simulink library "WECSim_Lib_Controllers"  (R2021b)
settings: Solver=ode45  StartTime=0.0  StopTime=10.0  RelTol=1e-3  EnableMultiTasking=on
undefined symbols (not defined in the file or in its folder): controller, controlSim, simu
settings Model: RequirementInfo="{}  %GIDa_42666abb_d6d9_408c_ae24_f6520282b61c"  Creator=sor  LastModifiedBy=jtgrasb
settings SolverCC: AlgebraicLoopSolver=TrustRegion
settings DataIOCC: LimitDataPoints=on  SaveFormat=Array  ReturnWorkspaceOutputs=off
settings OptimizationCC: LifeSpan=inf
settings DebuggingCC: SolverPrmCheckMsg=warning  AllowSymbolicDim=off  SFUnexpectedBacktrackingDiag=warning  SFNoUnconditionalDefaultTransitionDiag=warning  SFExecutionAtInitializationDiag=none  SFMachineParentedDataDiag=warning  ArithmeticOperatorsInVariantConditions=warning
settings HardwareCC: ProdBitPerPointer=32  ProdBitPerSizeT=32  ProdBitPerPtrDiffT=32  ProdLargestAtomicFloat=None  ProdIntDivRoundTo=Undefined  ProdEndianess=Unspecified  ProdWordSize=32  ProdHWDeviceType=32-bit Generic
settings ModelReferenceCC: PropagateSignalLabelsOutOfModel=off
settings SFSimCC: SimUseLocalCustomCode=off  CustomCodeUndefinedFunction=UseInterfaceOnly
settings RTWCC: RTWUseLocalCustomCode=off
settings CodeAppCC: StateflowObjectComments=on
settings GRTTargetCC: TargetLangStandard=C89/C90 (ANSI)
settings ConfigComp: CovMetricSettings=dw  CovSaveCumulativeToWorkspaceVar=on  CovSaveSingleToWorkspaceVar=on  CovExternalEMLEnable=off  CovSFcnEnable=off

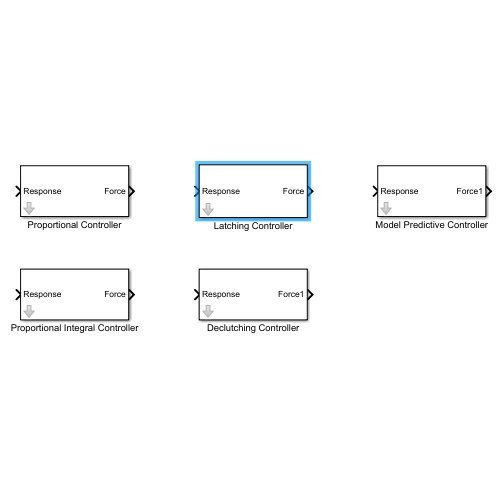
[thumbnail: Simulink's stored preview of the top-level diagram]
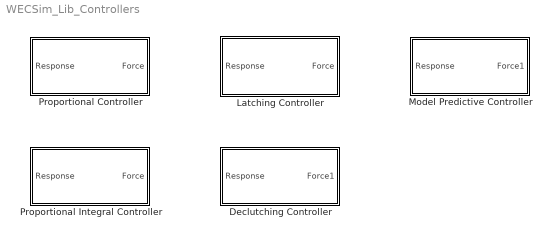
== system WECSim_Lib_Controllers ==
  Declutching Controller : Subsystem  mask{controller=controller(1), InputFiletext=Use WEC-Sim input file to define Latching Controller parameters, Kp=0, Ki=0, declutchTime=0}
      mask prompts: controller "Controller Name:"; Kp "Proportional gain (damping) [Ns/m]"; Ki "Integral gain (stiffness) [N/m]"; declutchTime "Declutching Time [s]"
      mask init:
      | if exist('controller','var')
      |     h=[gcb '/To Workspace'];
      |     responseName=['controller' num2str(controller.number) '_out'];
      |     set_param(h,'VariableName',responseName);
      | end
      | clear h responseName
      mask DialogControl InputFileGroup Prompt: Input File
      mask DialogControl CustomParameterGroup Prompt: Custom Parameters
      mask DialogControl DCParameters Prompt: Declutching Controller Parameters
  Latching Controller : Subsystem  mask{controller=controller(1), InputFiletext=Use WEC-Sim input file to define Latching Controller parameters, Kp=0, Ki=0, latchTime=0}
      mask prompts: controller "Controller Name"; Kp "Proportional gain (damping) [Ns/m]"; Ki "Integral gain (stiffness) [N/m]"; latchTime "Latching Time [s]"
      mask init:
      | if exist('controller','var')
      |     h=[gcb '/To Workspace'];
      |     responseName=['controller' num2str(controller.number) '_out'];
      |     set_param(h,'VariableName',responseName);
      | end
      | clear h responseName
      mask DialogControl InputFileGroup Prompt: Input File
      mask DialogControl CustomParameterGroup Prompt: Custom Parameters
      mask DialogControl LCParameters Prompt: Latching Controller Parameters
  Model Predictive Controller : Subsystem  mask{controller=controller(1), InputFiletext=Use WEC-Sim input file to define Latching Controller parameters, Kp=0, Ki=0, declutchTime=0}
      mask prompts: controller "Controller Name:"; Kp "Proportional gain (damping) [Ns/m]"; Ki "Integral gain (stiffness) [N/m]"; declutchTime "Declutching Time [s]"
      mask init:
      | if exist('controller','var')
      |     h=[gcb '/To Workspace'];
      |     responseName=['controller' num2str(controller.number) '_out'];
      |     set_param(h,'VariableName',responseName);
      | end
      | clear h responseName
      mask DialogControl InputFileGroup Prompt: Input File
      mask DialogControl CustomParameterGroup Prompt: Custom Parameters
      mask DialogControl DCParameters Prompt: Declutching Controller Parameters
  Proportional Controller : Subsystem  mask{controller=controller(1), InputFiletext=Use WEC-Sim input file to define Latching Controller parameters, Kp=0}
      mask prompts: controller "Controller Name:"; Kp "Proportional gain (damping) [Ns/m]"
      mask init:
      | if exist('controller','var')
      |     h=[gcb '/To Workspace'];
      |     responseName=['controller' num2str(controller.number) '_out'];
      |     set_param(h,'VariableName',responseName);
      | end
      | clear h responseName
      mask DialogControl InputFileGroup Prompt: Input File
      mask DialogControl CustomParameterGroup Prompt: Custom Parameters
      mask DialogControl PCParameters Prompt: Proportional Controller Parameters
  Proportional Integral Controller : Subsystem  mask{controller=controller(1), InputFiletext=Use WEC-Sim input file to define Latching Controller parameters, Kp=0, Ki=0}
      mask prompts: controller "Controller Name:"; Kp "Proportional gain (damping) [Ns/m]"; Ki "Integral gain (stiffness) [N/m]"
      mask init:
      | if exist('controller','var')
      |     h=[gcb '/To Workspace'];
      |     responseName=['controller' num2str(controller.number) '_out'];
      |     set_param(h,'VariableName',responseName);
      | end
      | clear h responseName
      mask DialogControl InputFileGroup Prompt: Input File
      mask DialogControl CustomParameterGroup Prompt: Custom Parameters
      mask DialogControl PICParameters Prompt: Proportional Integral Controller Parameters

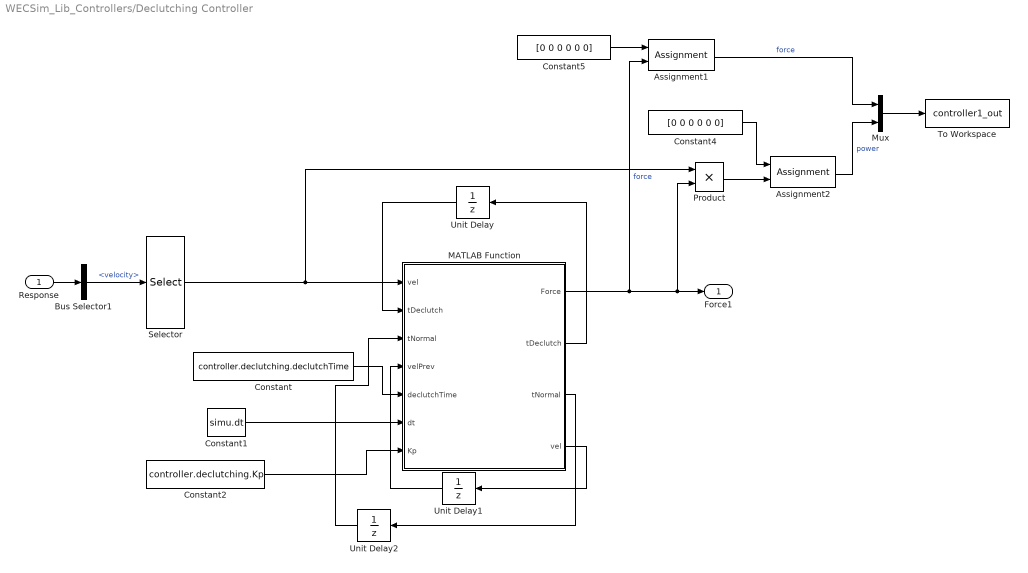
== system WECSim_Lib_Controllers/Declutching Controller ==
  Response : Inport
  Assignment1 : Assignment  IndexOptions=Index vector (dialog)  Indices=3  OutputSizes=1
  Assignment2 : Assignment  IndexOptions=Index vector (dialog)  Indices=3  OutputSizes=1
  Bus Selector1 : BusSelector  OutputSignals=velocity
  Constant : Constant  Value=controller.declutching.declutchTime
  Constant1 : Constant  Value=simu.dt
  Constant2 : Constant  Value=controller.declutching.Kp
  Constant4 : Constant  Value=[0 0 0 0 0 0]
  Constant5 : Constant  Value=[0 0 0 0 0 0]
  MATLAB Function : MATLAB Function  TreatAsAtomicUnit=on
  Mux : Mux  Inputs=2
  Product : Product
  Selector : Selector  InputPortWidth=6  IndexOptions=Index vector (dialog)  Indices=3  OutputSizes=1
  To Workspace : ToWorkspace  VariableName=controller1_out  SaveFormat=Structure With Time  SampleTime=simu.dtOut
  Unit Delay : UnitDelay  SampleTime=-1  HasFrameUpgradeWarning=on
  Unit Delay1 : UnitDelay  SampleTime=-1  HasFrameUpgradeWarning=on
  Unit Delay2 : UnitDelay  SampleTime=-1  HasFrameUpgradeWarning=on
  Force1 : Outport
  wires:
  Bus Selector1/1 -> Selector/1  "<velocity>"
  MATLAB Function/4(vel) -> Unit Delay1/1
  Unit Delay2/1 -> MATLAB Function/3("tNormal ")
  Constant2/1 -> MATLAB Function/7(Kp)
  Unit Delay1/1 -> MATLAB Function/4(velPrev)
  MATLAB Function/3(tNormal) -> Unit Delay2/1
  Constant/1 -> MATLAB Function/5(declutchTime)
  Unit Delay/1 -> MATLAB Function/2("tDeclutch ")
  Constant1/1 -> MATLAB Function/6(dt)
  MATLAB Function/2(tDeclutch) -> Unit Delay/1
  Response/1 -> Bus Selector1/1
  Constant4/1 -> Assignment2/1
  Assignment2/1 -> Mux/2  "power"
  Product/1 -> Assignment2/2
  MATLAB Function/1(Force) -> Force1/1, Product/2, Assignment1/2  "force"
  Assignment1/1 -> Mux/1  "force"
  Mux/1 -> To Workspace/1
  Selector/1 -> Product/1, MATLAB Function/1("vel ")
  Constant5/1 -> Assignment1/1

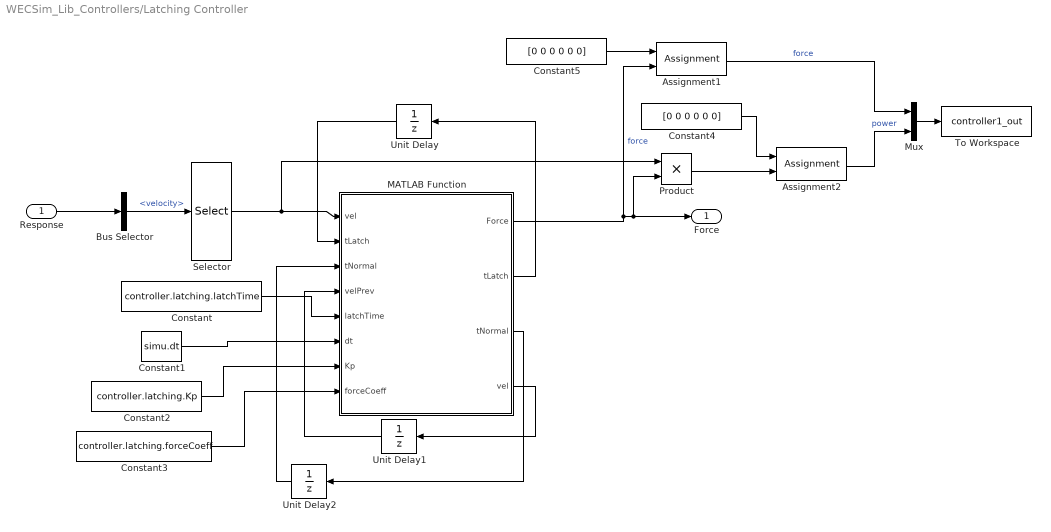
== system WECSim_Lib_Controllers/Latching Controller ==
  Response : Inport
  Assignment1 : Assignment  IndexOptions=Index vector (dialog)  Indices=3  OutputSizes=1
  Assignment2 : Assignment  IndexOptions=Index vector (dialog)  Indices=3  OutputSizes=1
  Bus Selector : BusSelector  OutputSignals=velocity
  Constant : Constant  Value=controller.latching.latchTime
  Constant1 : Constant  Value=simu.dt
  Constant2 : Constant  Value=controller.latching.Kp
  Constant3 : Constant  Value=controller.latching.forceCoeff
  Constant4 : Constant  Value=[0 0 0 0 0 0]
  Constant5 : Constant  Value=[0 0 0 0 0 0]
  MATLAB Function : MATLAB Function  TreatAsAtomicUnit=on
  Mux : Mux  Inputs=2
  Product : Product
  Selector : Selector  InputPortWidth=6  IndexOptions=Index vector (dialog)  Indices=3  OutputSizes=1
  To Workspace : ToWorkspace  VariableName=controller1_out  SaveFormat=Structure With Time  SampleTime=simu.dtOut
  Unit Delay : UnitDelay  SampleTime=-1  HasFrameUpgradeWarning=on
  Unit Delay1 : UnitDelay  SampleTime=-1  HasFrameUpgradeWarning=on
  Unit Delay2 : UnitDelay  SampleTime=-1  HasFrameUpgradeWarning=on
  Force : Outport
  wires:
  Constant1/1 -> MATLAB Function/6(dt)
  Response/1 -> Bus Selector/1
  MATLAB Function/3(tNormal) -> Unit Delay2/1
  MATLAB Function/2(tLatch) -> Unit Delay/1
  Unit Delay2/1 -> MATLAB Function/3("tNormal ")
  Unit Delay1/1 -> MATLAB Function/4(velPrev)
  Unit Delay/1 -> MATLAB Function/2("tLatch ")
  Bus Selector/1 -> Selector/1  "<velocity>"
  Constant/1 -> MATLAB Function/5(latchTime)
  Selector/1 -> Product/1, MATLAB Function/1("vel ")
  MATLAB Function/4(vel) -> Unit Delay1/1
  Constant2/1 -> MATLAB Function/7(Kp)
  Constant5/1 -> Assignment1/1
  Mux/1 -> To Workspace/1
  MATLAB Function/1(Force) -> Product/2, Force/1, Assignment1/2  "force"
  Assignment1/1 -> Mux/1  "force"
  Assignment2/1 -> Mux/2  "power"
  Product/1 -> Assignment2/2
  Constant4/1 -> Assignment2/1
  Constant3/1 -> MATLAB Function/8(forceCoeff)

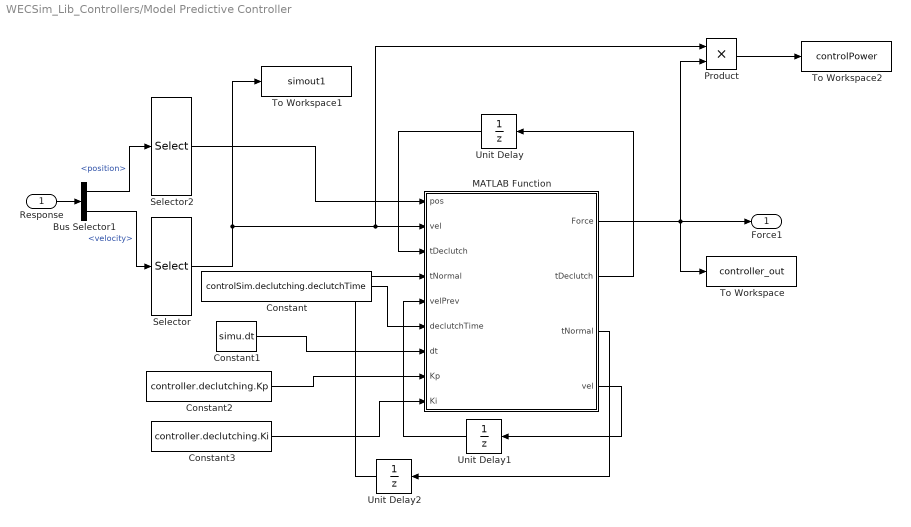
== system WECSim_Lib_Controllers/Model Predictive Controller ==
  Response : Inport
  Bus Selector1 : BusSelector  OutputSignals=position,velocity
  Constant : Constant  Value=controlSim.declutching.declutchTime
  Constant1 : Constant  Value=simu.dt
  Constant2 : Constant  Value=controller.declutching.Kp
  Constant3 : Constant  Value=controller.declutching.Ki
  MATLAB Function : MATLAB Function  TreatAsAtomicUnit=on
  Product : Product
  Selector : Selector  InputPortWidth=6  IndexOptions=Index vector (dialog)  Indices=3  OutputSizes=1
  Selector2 : Selector  InputPortWidth=6  IndexOptions=Index vector (dialog)  Indices=3  OutputSizes=1
  To Workspace : ToWorkspace  VariableName=controller_out  SaveFormat=Timeseries  SampleTime=-1
  To Workspace1 : ToWorkspace  VariableName=simout1  SaveFormat=Timeseries  SampleTime=-1
  To Workspace2 : ToWorkspace  VariableName=controlPower  SaveFormat=Timeseries  SampleTime=-1
  Unit Delay : UnitDelay  SampleTime=-1  HasFrameUpgradeWarning=on
  Unit Delay1 : UnitDelay  SampleTime=-1  HasFrameUpgradeWarning=on
  Unit Delay2 : UnitDelay  SampleTime=-1  HasFrameUpgradeWarning=on
  Force1 : Outport
  wires:
  Response/1 -> Bus Selector1/1
  MATLAB Function/2(tDeclutch) -> Unit Delay/1
  Constant1/1 -> MATLAB Function/7(dt)
  Unit Delay/1 -> MATLAB Function/3("tDeclutch ")
  Constant/1 -> MATLAB Function/6(declutchTime)
  MATLAB Function/3(tNormal) -> Unit Delay2/1
  Constant3/1 -> MATLAB Function/9(Ki)
  Unit Delay1/1 -> MATLAB Function/5(velPrev)
  Constant2/1 -> MATLAB Function/8(Kp)
  MATLAB Function/1(Force) -> To Workspace/1, Force1/1, Product/2
  Unit Delay2/1 -> MATLAB Function/4("tNormal ")
  MATLAB Function/4(vel) -> Unit Delay1/1
  Bus Selector1/2 -> Selector/1  "<velocity>"
  Selector/1 -> MATLAB Function/2("vel "), Product/1, To Workspace1/1
  Bus Selector1/1 -> Selector2/1  "<position>"
  Product/1 -> To Workspace2/1
  Selector2/1 -> MATLAB Function/1(pos)

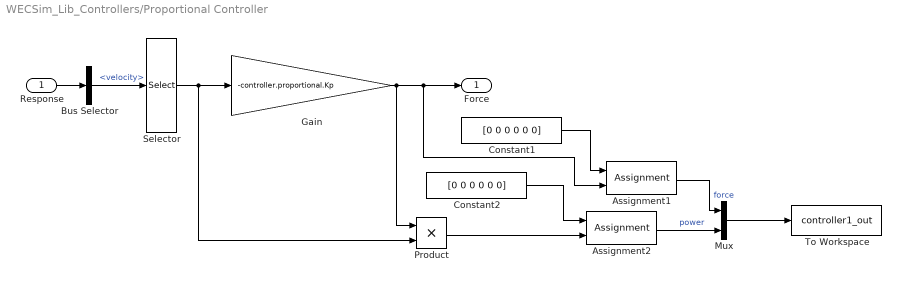
== system WECSim_Lib_Controllers/Proportional Controller ==
  Response : Inport
  Assignment1 : Assignment  IndexOptions=Index vector (dialog)  Indices=3  OutputSizes=1
  Assignment2 : Assignment  IndexOptions=Index vector (dialog)  Indices=3  OutputSizes=1
  Bus Selector : BusSelector  OutputSignals=velocity
  Constant1 : Constant  Value=[0 0 0 0 0 0]
  Constant2 : Constant  Value=[0 0 0 0 0 0]
  Gain : Gain  Gain=-controller.proportional.Kp
  Mux : Mux  Inputs=2
  Product : Product
  Selector : Selector  InputPortWidth=6  IndexOptions=Index vector (dialog)  Indices=3  OutputSizes=1
  To Workspace : ToWorkspace  VariableName=controller1_out  SaveFormat=Structure With Time  SampleTime=simu.dtOut
  Force : Outport
  wires:
  Gain/1 -> Product/1, Assignment1/2, Force/1
  Product/1 -> Assignment2/2
  Response/1 -> Bus Selector/1
  Bus Selector/1 -> Selector/1  "<velocity>"
  Mux/1 -> To Workspace/1
  Selector/1 -> Product/2, Gain/1
  Constant2/1 -> Assignment2/1
  Assignment2/1 -> Mux/2  "power"
  Constant1/1 -> Assignment1/1
  Assignment1/1 -> Mux/1  "force"

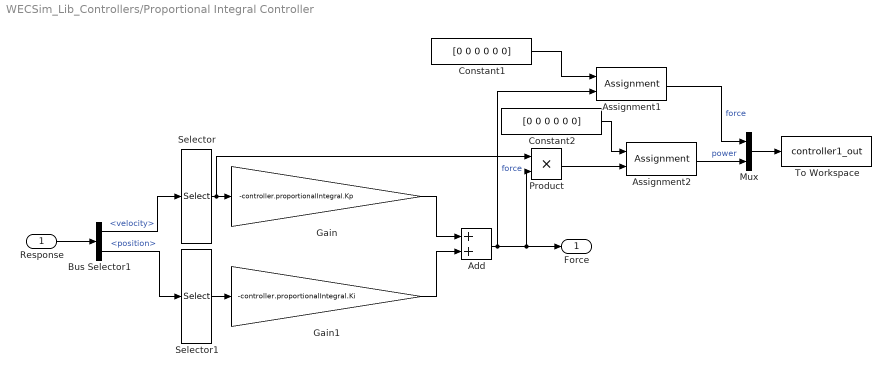
== system WECSim_Lib_Controllers/Proportional Integral Controller ==
  Response : Inport
  Add : Sum
  Assignment1 : Assignment  IndexOptions=Index vector (dialog)  Indices=3  OutputSizes=1
  Assignment2 : Assignment  IndexOptions=Index vector (dialog)  Indices=3  OutputSizes=1
  Bus Selector1 : BusSelector  OutputSignals=velocity,position
  Constant1 : Constant  Value=[0 0 0 0 0 0]
  Constant2 : Constant  Value=[0 0 0 0 0 0]
  Gain : Gain  Gain=-controller.proportionalIntegral.Kp
  Gain1 : Gain  Gain=-controller.proportionalIntegral.Ki
  Mux : Mux  Inputs=2
  Product : Product
  Selector : Selector  InputPortWidth=6  IndexOptions=Index vector (dialog)  Indices=3  OutputSizes=1
  Selector1 : Selector  InputPortWidth=6  IndexOptions=Index vector (dialog)  Indices=3  OutputSizes=1
  To Workspace : ToWorkspace  VariableName=controller1_out  SaveFormat=Structure With Time  SampleTime=simu.dtOut
  Force : Outport
  wires:
  Gain1/1 -> Add/2
  Add/1 -> Force/1, Product/2, Assignment1/2  "force"
  Gain/1 -> Add/1
  Response/1 -> Bus Selector1/1
  Bus Selector1/2 -> Selector1/1  "<position>"
  Mux/1 -> To Workspace/1
  Constant1/1 -> Assignment1/1
  Assignment2/1 -> Mux/2  "power"
  Assignment1/1 -> Mux/1  "force"
  Product/1 -> Assignment2/2
  Constant2/1 -> Assignment2/1
  Bus Selector1/1 -> Selector/1  "<velocity>"
  Selector/1 -> Product/1, Gain/1
  Selector1/1 -> Gain1/1

== matlab function WECSim_Lib_Controllers/Latching Controller/MATLAB Function ==
  data: vel input; Force output; tLatch input; tNormal input; velPrev input; tLatch output; tNormal output; vel output; latchTime input; dt input; Kp input; forceCoeff input
function [Force, tLatch, tNormal, vel] = latchingTime(vel, tLatch, tNormal, velPrev, latchTime, dt, Kp, forceCoeff)

[Force, tLatch, tNormal, vel] = latchingTime(vel, tLatch, tNormal, velPrev, latchTime, dt, Kp, forceCoeff);

end

== matlab function WECSim_Lib_Controllers/Declutching Controller/MATLAB Function ==
  data: vel input; Force output; tDeclutch input; tNormal input; velPrev input; tDeclutch output; tNormal output; vel output; declutchTime input; dt input; Kp input
function [Force, tDeclutch, tNormal, vel] = declutching(vel, tDeclutch, tNormal, velPrev, declutchTime, dt, Kp)

[Force, tDeclutch, tNormal, vel] = declutching(vel, tDeclutch, tNormal, velPrev, declutchTime, dt, Kp);

end

== matlab function WECSim_Lib_Controllers/Model Predictive Controller/MATLAB Function ==
  data: pos input; vel input; Force output; tDeclutch input; tNormal input; velPrev input; tDeclutch output; tNormal output; vel output; declutchTime input; dt input; Kp input; Ki input
function [Force, tDeclutch, tNormal, vel] = fcn(pos, vel, tDeclutch, tNormal, velPrev, declutchTime, dt, Kp, Ki)

if ((diff(sign([vel,velPrev]))~=0 && tDeclutch==0 && tNormal>.2) || (tDeclutch>0 && tDeclutch<declutchTime))
    Force = 0;
    tDeclutch = tDeclutch + dt;
    tNormal = 0;
else
    Force = -Kp*vel + -Ki*pos;
    tNormal = tNormal + dt;
    tDeclutch = 0;
end
end
